simulink model "BrakingHydraulics"  (R2026b)
settings: Solver=VariableStepAuto
undefined symbols (not defined in the file): PlntBrkFrntBias, PlntBrkPrsFctr, PlntBrkRearBias, PlntBrkWc
settings Model: ModifiedByFormat=The MathWorks, Inc.  Creator=The MathWorks, Inc.  LastModifiedBy=The MathWorks, Inc.
settings OptimizationCC: ReuseModelBlockBuffer=off

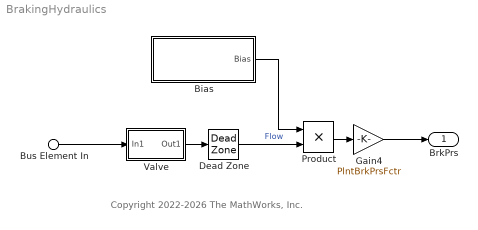
== system BrakingHydraulics ==
  note: Copyright 2022-2026 The MathWorks, Inc.
  Bus Element In : Inport  PortName=Cntrl  Element=Vcu.VcuBrkPrsCmd
  Bias : Subsystem  Variant=on  VariantControlMode=label  LabelModeActiveChoice=TwoAxleBraking
  Dead Zone : DeadZone  LowerValue=-inf  UpperValue=1e-3  ZeroCross=off
  Gain4 : Gain  Gain=PlntBrkPrsFctr
  Product : Product
  Valve : Subsystem  TreatAsAtomicUnit=on
  BrkPrs : Outport  VectorParamsAs1DForOutWhenUnconnected=off
  wires:
  Bias/1(Bias) -> Product/1
  Bus Element In/1 -> Valve/1(In1)
  Product/1 -> Gain4/1
  Dead Zone/1 -> Product/2  "Flow"
  Gain4/1 -> BrkPrs/1
  Valve/1(Out1) -> Dead Zone/1

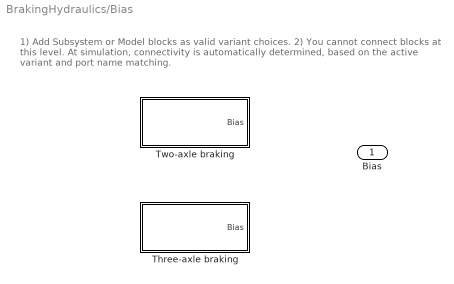
== system BrakingHydraulics/Bias ==
  note: 1) Add Subsystem or Model blocks as valid variant choices.
      | 2) You cannot connect blocks at this level. At simulation, connectivity is automatically
      | determined, based on the active variant and port name matching.
  Three-axle braking : Subsystem  VariantControl=ThreeAxleBraking
  Two-axle braking : Subsystem  VariantControl=TwoAxleBraking
  Bias : Outport

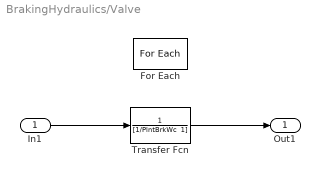
== system BrakingHydraulics/Valve ==
  In1 : Inport  Partition=on  PartitionDimension=1  PartitionWidth=1  PartitionOffset=0
  For Each : ForEach  DisableCoverage=on
  Transfer Fcn : TransferFcn  Denominator="[1/PlntBrkWc  1]"
  Out1 : Outport  ConcatenationDimension=1
  wires:
  In1/1 -> Transfer Fcn/1
  Transfer Fcn/1 -> Out1/1

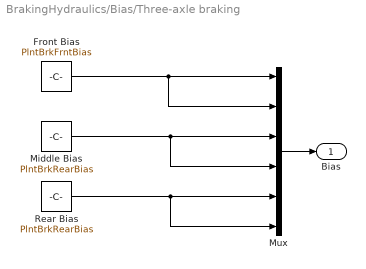
== system BrakingHydraulics/Bias/Three-axle braking ==
  Front Bias : Constant  Value=PlntBrkFrntBias  SampleTime=-1
  Middle Bias : Constant  Value=PlntBrkRearBias  SampleTime=-1
  Mux : Mux  Inputs=6
  Rear Bias : Constant  Value=PlntBrkRearBias  SampleTime=-1
  Bias : Outport
  wires:
  Rear Bias/1 -> Mux/6, Mux/5
  Front Bias/1 -> Mux/2, Mux/1
  Mux/1 -> Bias/1
  Middle Bias/1 -> Mux/4, Mux/3

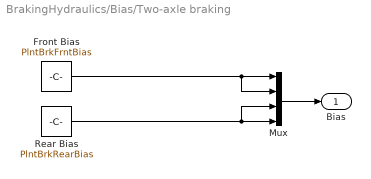
== system BrakingHydraulics/Bias/Two-axle braking ==
  Front Bias : Constant  Value=PlntBrkFrntBias  SampleTime=-1
  Mux : Mux
  Rear Bias : Constant  Value=PlntBrkRearBias  SampleTime=-1
  Bias : Outport
  wires:
  Rear Bias/1 -> Mux/3, Mux/4
  Front Bias/1 -> Mux/2, Mux/1
  Mux/1 -> Bias/1
